simulink model "ThermalTank_Controller"  (R2023a)
settings: Solver=ode4  StartTime=0.0  StopTime=8  FixedStep=0.001  RelTol=1e-3
settings Model: Creator=Fasih  LastModifiedBy=Fasih

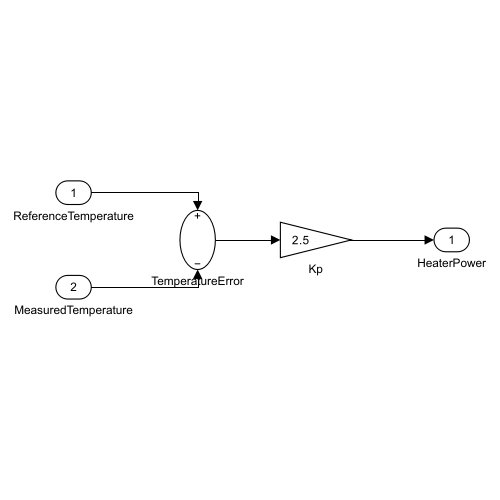
[thumbnail: Simulink's stored preview of the top-level diagram]
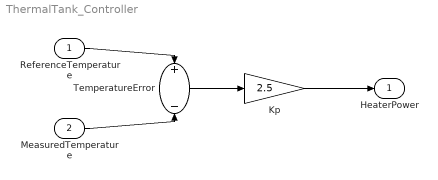
== system ThermalTank_Controller ==
  ReferenceTemperature : Inport
  MeasuredTemperature : Inport  Port=2
  Kp : Gain  Gain=2.5
  TemperatureError : Sum  Inputs=+-
  HeaterPower : Outport
  wires:
  ReferenceTemperature/1 -> TemperatureError/1
  MeasuredTemperature/1 -> TemperatureError/2
  TemperatureError/1 -> Kp/1
  Kp/1 -> HeaterPower/1
